simulink model "mrefrobotarm_modified_previous_y_previous_u_previous_ref_Thao"  (R2018b)
settings: Solver=FixedStepAuto  StartTime=0.0  StopTime=10  RelTol=1e-3  AbsTol=1e-6
undefined symbols (not defined in the file or in its folder): sfunxy2
libraries: neural x668, simulink x1
(part 21 of 21)

== system mrefrobotarm_modified_previous_y_previous_u_previous_ref_Thao/working_test/Layer 2/LW{2,1} ==
  "ad{2,1}" : Inport  PortDimensions=8
      mask Display: e = 0.06;c1 = [120 230 180]/255;c2 = ([120 230 180]+0)/(256+128);c3 = ([120 230 180]+128)/(256+128);patch([0 1 1 0],[0 0 1 1],c1);patch([0 1 1 1-e 1-e 0+e],[0 0 1 1-e 0+e 0+e],c2);patch([0 0 1 1-e 0+e 0+e],[0 1 1 1-e 1-e 0+e],c3);plot([0 1 1 0 0],[0 0 1 1 0]);
  "IW{2,1}(1,:)'" : Constant  Value=[1.463550825562915935762475783121772110462188720703125;1.2082669866689801363435208259033970534801483154296875;-0.6229993629461720860973628077772445976734161376953125;0.488116211879852102129007107578217983245849609375;0.84588482114214647022976123480475507676601409912109375;-1.1928719541486427768717248909524641931056976318359375;-2.057825620782761877336497491342015564441680908203125;1.5399555707144136906805442777113057672977447509765625]
      mask Display: e = 0.06;c1 = [120 150 230]/255;c2 = ([120 150 230]+0)/383;c3 = ([120 150 230]+128)/383;patch([0 1 1 0],[0 0 1 1],c1);patch([0 1 1 1-e 1-e 0+e],[0 0 1 1-e 0+e 0+e],c2);patch([0 0 1 1-e 0+e 0+e],[0 1 1 1-e 1-e 0+e],c3);plot([0 1 1 0 0],[0 0 1 1 0]);disp('weights');
  "IW{2,1}(10,:)'" : Constant  Value=[1.134018666679956321985400791163556277751922607421875;0.99363946648308232312274412834085524082183837890625;-0.54676888111817933957325976734864525496959686279296875;-0.76340597417966515880749511779868043959140777587890625;-0.9815147483076629431053561347653158009052276611328125;0.5968332702765632991059874257189221680164337158203125;1.9952854954885268501385553463478572666645050048828125;-0.92110586776434277833658370582270435988903045654296875]
      mask Display: e = 0.06;c1 = [120 150 230]/255;c2 = ([120 150 230]+0)/383;c3 = ([120 150 230]+128)/383;patch([0 1 1 0],[0 0 1 1],c1);patch([0 1 1 1-e 1-e 0+e],[0 0 1 1-e 0+e 0+e],c2);patch([0 0 1 1-e 0+e 0+e],[0 1 1 1-e 1-e 0+e],c3);plot([0 1 1 0 0],[0 0 1 1 0]);disp('weights');
  "IW{2,1}(11,:)'" : Constant  Value=[0.434041573917725853615223741144291125237941741943359375;0.16471617384395731420454467297531664371490478515625;-0.216118041022805462691991351675824262201786041259765625;2.8978280304609853601505164988338947296142578125;1.943598394902243509108075159019790589809417724609375;4.6129183278583578697862321860156953334808349609375;-0.81063433781615701345657498677610419690608978271484375;1.7612531272589067032896537057240493595600128173828125]
      mask Display: e = 0.06;c1 = [120 150 230]/255;c2 = ([120 150 230]+0)/383;c3 = ([120 150 230]+128)/383;patch([0 1 1 0],[0 0 1 1],c1);patch([0 1 1 1-e 1-e 0+e],[0 0 1 1-e 0+e 0+e],c2);patch([0 0 1 1-e 0+e 0+e],[0 1 1 1-e 1-e 0+e],c3);plot([0 1 1 0 0],[0 0 1 1 0]);disp('weights');
  "IW{2,1}(12,:)'" : Constant  Value=[1.74376096782253586781052945298142731189727783203125;0.94016947729569444458519456020439974963665008544921875;0.773288113770950413794480482465587556362152099609375;-0.72054867623120422148730312983389012515544891357421875;-0.06420804673181064459175360070730675943195819854736328125;-1.447472796373246328727191212237812578678131103515625;-0.06982005075191678733492750552613870240747928619384765625;1.6685199899347125107595957160810939967632293701171875]
      mask Display: e = 0.06;c1 = [120 150 230]/255;c2 = ([120 150 230]+0)/383;c3 = ([120 150 230]+128)/383;patch([0 1 1 0],[0 0 1 1],c1);patch([0 1 1 1-e 1-e 0+e],[0 0 1 1-e 0+e 0+e],c2);patch([0 0 1 1-e 0+e 0+e],[0 1 1 1-e 1-e 0+e],c3);plot([0 1 1 0 0],[0 0 1 1 0]);disp('weights');
  "IW{2,1}(13,:)'" : Constant  Value=[0.58611133181064423158801446334109641611576080322265625;-2.424919354117549108451612482895143330097198486328125;0.275534914445166367880091229380923323333263397216796875;-0.3179661163902725018459705097484402358531951904296875;-0.3847035616320677586799092750879935920238494873046875;-0.63707268499747760071016955407685600221157073974609375;-0.260138967832102441235520018381066620349884033203125;1.4313466678042507940205041450099088251590728759765625]
      mask Display: e = 0.06;c1 = [120 150 230]/255;c2 = ([120 150 230]+0)/383;c3 = ([120 150 230]+128)/383;patch([0 1 1 0],[0 0 1 1],c1);patch([0 1 1 1-e 1-e 0+e],[0 0 1 1-e 0+e 0+e],c2);patch([0 0 1 1-e 0+e 0+e],[0 1 1 1-e 1-e 0+e],c3);plot([0 1 1 0 0],[0 0 1 1 0]);disp('weights');
  "IW{2,1}(14,:)'" : Constant  Value=[-0.1330838655979345308555394922223058529198169708251953125;0.0807940849429321372721091165658435784280300140380859375;0.04937131990086006394502504690535715781152248382568359375;0.1369701045960752538999116723061888478696346282958984375;0.362315967016541840006738084412063471972942352294921875;0.2007900692008469933913517024848260916769504547119140625;0.357746870703516017808709648306830786168575286865234375;-1.0009625334190765943986889396910555660724639892578125]
      mask Display: e = 0.06;c1 = [120 150 230]/255;c2 = ([120 150 230]+0)/383;c3 = ([120 150 230]+128)/383;patch([0 1 1 0],[0 0 1 1],c1);patch([0 1 1 1-e 1-e 0+e],[0 0 1 1-e 0+e 0+e],c2);patch([0 0 1 1-e 0+e 0+e],[0 1 1 1-e 1-e 0+e],c3);plot([0 1 1 0 0],[0 0 1 1 0]);disp('weights');
  "IW{2,1}(15,:)'" : Constant  Value=[-1.5828584005342116736159141510142944753170013427734375;-0.34671511698060231143614373650052584707736968994140625;-0.208261551930768173956920463751885108649730682373046875;-0.71627429917518081747829228334012441337108612060546875;-1.3986327814857142382010124492808245122432708740234375;-0.033035758090816567944525417033219127915799617767333984375;1.820729591401267111194783865357749164104461669921875;-0.698698176789807501307905113208107650279998779296875]
      mask Display: e = 0.06;c1 = [120 150 230]/255;c2 = ([120 150 230]+0)/383;c3 = ([120 150 230]+128)/383;patch([0 1 1 0],[0 0 1 1],c1);patch([0 1 1 1-e 1-e 0+e],[0 0 1 1-e 0+e 0+e],c2);patch([0 0 1 1-e 0+e 0+e],[0 1 1 1-e 1-e 0+e],c3);plot([0 1 1 0 0],[0 0 1 1 0]);disp('weights');
  "IW{2,1}(16,:)'" : Constant  Value=[-1.5424575787334042775711395734106190502643585205078125;0.480620712648137493605560166543000377714633941650390625;-0.257424583228552383840082029564655385911464691162109375;-0.388965205406854419578621673281304538249969482421875;-1.523713504572799859460019433754496276378631591796875;0.39055994618596445722147336709895171225070953369140625;-2.445046000285369558469028561376035213470458984375;-1.9333998277230464157838696337421424686908721923828125]
      mask Display: e = 0.06;c1 = [120 150 230]/255;c2 = ([120 150 230]+0)/383;c3 = ([120 150 230]+128)/383;patch([0 1 1 0],[0 0 1 1],c1);patch([0 1 1 1-e 1-e 0+e],[0 0 1 1-e 0+e 0+e],c2);patch([0 0 1 1-e 0+e 0+e],[0 1 1 1-e 1-e 0+e],c3);plot([0 1 1 0 0],[0 0 1 1 0]);disp('weights');
  "IW{2,1}(17,:)'" : Constant  Value=[1.9202741200888648887001863840851001441478729248046875;3.59469018792837946563167861313559114933013916015625;1.278669491064107877065225693513639271259307861328125;0.1419885423222841669410598797185230068862438201904296875;-1.761399045758413439699552327510900795459747314453125;0.77646861010138745751163469321909360587596893310546875;-1.5057318919463986706119840164319612085819244384765625;4.2090514522541706554648044402711093425750732421875]
      mask Display: e = 0.06;c1 = [120 150 230]/255;c2 = ([120 150 230]+0)/383;c3 = ([120 150 230]+128)/383;patch([0 1 1 0],[0 0 1 1],c1);patch([0 1 1 1-e 1-e 0+e],[0 0 1 1-e 0+e 0+e],c2);patch([0 0 1 1-e 0+e 0+e],[0 1 1 1-e 1-e 0+e],c3);plot([0 1 1 0 0],[0 0 1 1 0]);disp('weights');
  "IW{2,1}(18,:)'" : Constant  Value=[2.24640861704423056011137305176816880702972412109375;0.53203674056552296978139793282025493681430816650390625;2.1547296277043468393230796209536492824554443359375;-0.9815123424716112321419814179535023868083953857421875;-0.95472145497063853891717144506401382386684417724609375;1.98605895577709556931722545414231717586517333984375;-0.034412853847981296484537239166456856764853000640869140625;5.09817173012213498139999501290731132030487060546875]
      mask Display: e = 0.06;c1 = [120 150 230]/255;c2 = ([120 150 230]+0)/383;c3 = ([120 150 230]+128)/383;patch([0 1 1 0],[0 0 1 1],c1);patch([0 1 1 1-e 1-e 0+e],[0 0 1 1-e 0+e 0+e],c2);patch([0 0 1 1-e 0+e 0+e],[0 1 1 1-e 1-e 0+e],c3);plot([0 1 1 0 0],[0 0 1 1 0]);disp('weights');
  "IW{2,1}(19,:)'" : Constant  Value=[0.7794520854145703392390487351804040372371673583984375;-1.895929436985962279749173831078223884105682373046875;-1.7189894476246034837885190427186898887157440185546875;-0.6837047167167085159888983980636112391948699951171875;0.34353814452782016619636351606459356844425201416015625;-4.143145140083309030387681559659540653228759765625;2.2429389993183068696680493303574621677398681640625;3.682068418408167786992635228671133518218994140625]
      mask Display: e = 0.06;c1 = [120 150 230]/255;c2 = ([120 150 230]+0)/383;c3 = ([120 150 230]+128)/383;patch([0 1 1 0],[0 0 1 1],c1);patch([0 1 1 1-e 1-e 0+e],[0 0 1 1-e 0+e 0+e],c2);patch([0 0 1 1-e 0+e 0+e],[0 1 1 1-e 1-e 0+e],c3);plot([0 1 1 0 0],[0 0 1 1 0]);disp('weights');
  "IW{2,1}(2,:)'" : Constant  Value=[1.0654566777175968894653124152682721614837646484375;0.002032816601710635100175306178016398916952311992645263671875;2.1595672663571736649146259878762066364288330078125;0.92280763301808221843458568400819785892963409423828125;1.768096961470302375118990312330424785614013671875;1.6041779041884136614015687882783822715282440185546875;0.7628890513396715533644965034909546375274658203125;-3.6541749563162664315996153163723647594451904296875]
      mask Display: e = 0.06;c1 = [120 150 230]/255;c2 = ([120 150 230]+0)/383;c3 = ([120 150 230]+128)/383;patch([0 1 1 0],[0 0 1 1],c1);patch([0 1 1 1-e 1-e 0+e],[0 0 1 1-e 0+e 0+e],c2);patch([0 0 1 1-e 0+e 0+e],[0 1 1 1-e 1-e 0+e],c3);plot([0 1 1 0 0],[0 0 1 1 0]);disp('weights');
  "IW{2,1}(20,:)'" : Constant  Value=[-0.103154969350188807641899302325327880680561065673828125;2.252970323340981462223453490878455340862274169921875;-0.96843329729804239480728256239672191441059112548828125;-1.902193396943337777571514379815198481082916259765625;0.366418820839169268044344107693177647888660430908203125;-2.270850899561910551938126445747911930084228515625;-1.3039885334908654090924073898349888622760772705078125;0.50925510859634848248589378272299654781818389892578125]
      mask Display: e = 0.06;c1 = [120 150 230]/255;c2 = ([120 150 230]+0)/383;c3 = ([120 150 230]+128)/383;patch([0 1 1 0],[0 0 1 1],c1);patch([0 1 1 1-e 1-e 0+e],[0 0 1 1-e 0+e 0+e],c2);patch([0 0 1 1-e 0+e 0+e],[0 1 1 1-e 1-e 0+e],c3);plot([0 1 1 0 0],[0 0 1 1 0]);disp('weights');
  "IW{2,1}(3,:)'" : Constant  Value=[-0.66339214473495022872384652146138250827789306640625;-0.222233047173612863200986566880601458251476287841796875;-0.81637664684851396490472552613937295973300933837890625;-0.668398882047606779366333284997381269931793212890625;1.9962758949163597055331820229184813797473907470703125;-0.27992544835338295516891093939193524420261383056640625;-0.94498420997124610298811830944032408297061920166015625;0.337485237137902682746926075196824967861175537109375]
      mask Display: e = 0.06;c1 = [120 150 230]/255;c2 = ([120 150 230]+0)/383;c3 = ([120 150 230]+128)/383;patch([0 1 1 0],[0 0 1 1],c1);patch([0 1 1 1-e 1-e 0+e],[0 0 1 1-e 0+e 0+e],c2);patch([0 0 1 1-e 0+e 0+e],[0 1 1 1-e 1-e 0+e],c3);plot([0 1 1 0 0],[0 0 1 1 0]);disp('weights');
  "IW{2,1}(4,:)'" : Constant  Value=[-2.20465810888284341473308813874609768390655517578125;2.584547994441787732711190983536653220653533935546875;-1.0462844726166229403219176674610935151576995849609375;3.5487772443023413160290147061459720134735107421875;-0.182806955450451835698544300612411461770534515380859375;0.235620634411733476110129004155169241130352020263671875;-2.22555439962967671618798704002983868122100830078125;-2.11305052916475322177802809164859354496002197265625]
      mask Display: e = 0.06;c1 = [120 150 230]/255;c2 = ([120 150 230]+0)/383;c3 = ([120 150 230]+128)/383;patch([0 1 1 0],[0 0 1 1],c1);patch([0 1 1 1-e 1-e 0+e],[0 0 1 1-e 0+e 0+e],c2);patch([0 0 1 1-e 0+e 0+e],[0 1 1 1-e 1-e 0+e],c3);plot([0 1 1 0 0],[0 0 1 1 0]);disp('weights');
  "IW{2,1}(5,:)'" : Constant  Value=[1.31774560984433275478977520833723247051239013671875;-0.360000305828590716483716960283345542848110198974609375;-0.311464151704573255496910633155493997037410736083984375;-1.0610633589393507758558143905247561633586883544921875;0.6481786802746196674007705951225943863391876220703125;1.9720589174498897033771527276257984340190887451171875;0.7658460266185020959284202035632915794849395751953125;3.26223001214720564888693843386135995388031005859375]
      mask Display: e = 0.06;c1 = [120 150 230]/255;c2 = ([120 150 230]+0)/383;c3 = ([120 150 230]+128)/383;patch([0 1 1 0],[0 0 1 1],c1);patch([0 1 1 1-e 1-e 0+e],[0 0 1 1-e 0+e 0+e],c2);patch([0 0 1 1-e 0+e 0+e],[0 1 1 1-e 1-e 0+e],c3);plot([0 1 1 0 0],[0 0 1 1 0]);disp('weights');
  "IW{2,1}(6,:)'" : Constant  Value=[0.7726601955585319370101160529884509742259979248046875;0.58889404743400375341622066116542555391788482666015625;-1.0756676160532527841695582537795417010784149169921875;-1.197073377238570213165758104878477752208709716796875;0.030446979813859798014163970947265625;-0.4042833226405779800671780321863479912281036376953125;0.42715808275051048159554056837805546820163726806640625;-0.6995334276770768244801956825540401041507720947265625]
      mask Display: e = 0.06;c1 = [120 150 230]/255;c2 = ([120 150 230]+0)/383;c3 = ([120 150 230]+128)/383;patch([0 1 1 0],[0 0 1 1],c1);patch([0 1 1 1-e 1-e 0+e],[0 0 1 1-e 0+e 0+e],c2);patch([0 0 1 1-e 0+e 0+e],[0 1 1 1-e 1-e 0+e],c3);plot([0 1 1 0 0],[0 0 1 1 0]);disp('weights');
  "IW{2,1}(7,:)'" : Constant  Value=[-0.7725295931807278915215420056483708322048187255859375;-2.173121115889052656910962468828074634075164794921875;-0.1818589726845724896531208969463477842509746551513671875;0.637043349560801441811008771765045821666717529296875;-2.165436289512435497073283841018564999103546142578125;2.37097135712689777164996485225856304168701171875;2.277406878831848668909287880524061620235443115234375;-1.4636931671188297965358060537255369126796722412109375]
      mask Display: e = 0.06;c1 = [120 150 230]/255;c2 = ([120 150 230]+0)/383;c3 = ([120 150 230]+128)/383;patch([0 1 1 0],[0 0 1 1],c1);patch([0 1 1 1-e 1-e 0+e],[0 0 1 1-e 0+e 0+e],c2);patch([0 0 1 1-e 0+e 0+e],[0 1 1 1-e 1-e 0+e],c3);plot([0 1 1 0 0],[0 0 1 1 0]);disp('weights');
  "IW{2,1}(8,:)'" : Constant  Value=[2.6381111188624846164429982309229671955108642578125;2.13100131299981665478071590769104659557342529296875;-1.6010659213930111821611035338719375431537628173828125;-0.046612756831267587731559842723072506487369537353515625;1.1429029499162701721814983102376572787761688232421875;-0.6486750417208211327846356653026305139064788818359375;1.9735437620485793974722810162347741425037384033203125;1.296947831419701824273715828894637525081634521484375]
      mask Display: e = 0.06;c1 = [120 150 230]/255;c2 = ([120 150 230]+0)/383;c3 = ([120 150 230]+128)/383;patch([0 1 1 0],[0 0 1 1],c1);patch([0 1 1 1-e 1-e 0+e],[0 0 1 1-e 0+e 0+e],c2);patch([0 0 1 1-e 0+e 0+e],[0 1 1 1-e 1-e 0+e],c3);plot([0 1 1 0 0],[0 0 1 1 0]);disp('weights');
  "IW{2,1}(9,:)'" : Constant  Value=[0.389378863511709749634093213899177499115467071533203125;-3.044010638669162549518887317390181124210357666015625;2.170328036093251089511113605112768709659576416015625;3.090312720034663840351640828885138034820556640625;-1.84388163895774592759835286415182054042816162109375;-0.35509810169707411997563895056373439729213714599609375;-2.31952597061908960540677071548998355865478515625;-1.2086983328395906056584863108582794666290283203125]
      mask Display: e = 0.06;c1 = [120 150 230]/255;c2 = ([120 150 230]+0)/383;c3 = ([120 150 230]+128)/383;patch([0 1 1 0],[0 0 1 1],c1);patch([0 1 1 1-e 1-e 0+e],[0 0 1 1-e 0+e 0+e],c2);patch([0 0 1 1-e 0+e 0+e],[0 1 1 1-e 1-e 0+e],c3);plot([0 1 1 0 0],[0 0 1 1 0]);disp('weights');
  Mux : Mux  Inputs=20
      mask Display: e = 0.06;c1 = [120 150 230]/255;c2 = ([120 150 230]+0)/383;c3 = ([120 150 230]+128)/383;patch([0 1 1 0],[0 0 1 1],c1);patch([0 1 1 1-e 1-e 0+e],[0 0 1 1-e 0+e 0+e],c2);patch([0 0 1 1-e 0+e 0+e],[0 1 1 1-e 1-e 0+e],c3);plot([0 1 1 0 0],[0 0 1 1 0]);disp('Mux');
  dotprod{1..20} (20 alike) : neural/Weight Functions/dotprod
  "lz{2,1}" : Outport
      mask Display: e = 0.06;c1 = [120 230 180]/255;c2 = ([120 230 180]+0)/(256+128);c3 = ([120 230 180]+128)/(256+128);patch([0 1 1 0],[0 0 1 1],c1);patch([0 1 1 1-e 1-e 0+e],[0 0 1 1-e 0+e 0+e],c2);patch([0 0 1 1-e 0+e 0+e],[0 1 1 1-e 1-e 0+e],c3);plot([0 1 1 0 0],[0 0 1 1 0]);
  wires:
  "IW{2,1}(1,:)'"/1 -> dotprod1/1
  "ad{2,1}"/1 -> dotprod1/2, dotprod2/2, dotprod3/2, dotprod4/2, dotprod5/2, dotprod6/2, dotprod7/2, dotprod8/2, dotprod9/2, dotprod10/2, dotprod11/2, dotprod12/2, dotprod13/2, dotprod14/2, dotprod15/2, dotprod16/2, dotprod17/2, dotprod18/2, dotprod19/2, dotprod20/2
  dotprod1/1 -> Mux/1
  "IW{2,1}(2,:)'"/1 -> dotprod2/1
  dotprod2/1 -> Mux/2
  "IW{2,1}(3,:)'"/1 -> dotprod3/1
  dotprod3/1 -> Mux/3
  "IW{2,1}(4,:)'"/1 -> dotprod4/1
  dotprod4/1 -> Mux/4
  "IW{2,1}(5,:)'"/1 -> dotprod5/1
  dotprod5/1 -> Mux/5
  "IW{2,1}(6,:)'"/1 -> dotprod6/1
  dotprod6/1 -> Mux/6
  "IW{2,1}(7,:)'"/1 -> dotprod7/1
  dotprod7/1 -> Mux/7
  "IW{2,1}(8,:)'"/1 -> dotprod8/1
  dotprod8/1 -> Mux/8
  "IW{2,1}(9,:)'"/1 -> dotprod9/1
  dotprod9/1 -> Mux/9
  "IW{2,1}(10,:)'"/1 -> dotprod10/1
  dotprod10/1 -> Mux/10
  "IW{2,1}(11,:)'"/1 -> dotprod11/1
  dotprod11/1 -> Mux/11
  "IW{2,1}(12,:)'"/1 -> dotprod12/1
  dotprod12/1 -> Mux/12
  "IW{2,1}(13,:)'"/1 -> dotprod13/1
  dotprod13/1 -> Mux/13
  "IW{2,1}(14,:)'"/1 -> dotprod14/1
  dotprod14/1 -> Mux/14
  "IW{2,1}(15,:)'"/1 -> dotprod15/1
  dotprod15/1 -> Mux/15
  "IW{2,1}(16,:)'"/1 -> dotprod16/1
  dotprod16/1 -> Mux/16
  "IW{2,1}(17,:)'"/1 -> dotprod17/1
  dotprod17/1 -> Mux/17
  "IW{2,1}(18,:)'"/1 -> dotprod18/1
  dotprod18/1 -> Mux/18
  "IW{2,1}(19,:)'"/1 -> dotprod19/1
  dotprod19/1 -> Mux/19
  "IW{2,1}(20,:)'"/1 -> dotprod20/1
  dotprod20/1 -> Mux/20
  Mux/1 -> "lz{2,1}"/1

== system mrefrobotarm_modified_previous_y_previous_u_previous_ref_Thao/working_test/Layer 3/Delays 1 ==
  "p{3}" : Inport  PortDimensions=20
      mask Display: e = 0.06;c1 = [120 230 180]/255;c2 = ([120 230 180]+0)/(256+128);c3 = ([120 230 180]+128)/(256+128);patch([0 1 1 0],[0 0 1 1],c1);patch([0 1 1 1-e 1-e 0+e],[0 0 1 1-e 0+e 0+e],c2);patch([0 0 1 1-e 0+e 0+e],[0 1 1 1-e 1-e 0+e],c3);plot([0 1 1 0 0],[0 0 1 1 0]);
  mux : Mux  Inputs=1
      mask Display: e = 0.06;c1 = [120 150 230]/255;c2 = ([120 150 230]+0)/383;c3 = ([120 150 230]+128)/383;patch([0 1 1 0],[0 0 1 1],c1);patch([0 1 1 1-e 1-e 0+e],[0 0 1 1-e 0+e 0+e],c2);patch([0 0 1 1-e 0+e 0+e],[0 1 1 1-e 1-e 0+e],c3);plot([0 1 1 0 0],[0 0 1 1 0]);disp('Mux')
  "pd{3,2}" : Outport
      mask Display: e = 0.06;c1 = [120 230 180]/255;c2 = ([120 230 180]+0)/(256+128);c3 = ([120 230 180]+128)/(256+128);patch([0 1 1 0],[0 0 1 1],c1);patch([0 1 1 1-e 1-e 0+e],[0 0 1 1-e 0+e 0+e],c2);patch([0 0 1 1-e 0+e 0+e],[0 1 1 1-e 1-e 0+e],c3);plot([0 1 1 0 0],[0 0 1 1 0]);
  wires:
  "p{3}"/1 -> mux/1
  mux/1 -> "pd{3,2}"/1

== system mrefrobotarm_modified_previous_y_previous_u_previous_ref_Thao/working_test/Layer 3/LW{3,2} ==
  "ad{3,2}" : Inport  PortDimensions=20
      mask Display: e = 0.06;c1 = [120 230 180]/255;c2 = ([120 230 180]+0)/(256+128);c3 = ([120 230 180]+128)/(256+128);patch([0 1 1 0],[0 0 1 1],c1);patch([0 1 1 1-e 1-e 0+e],[0 0 1 1-e 0+e 0+e],c2);patch([0 0 1 1-e 0+e 0+e],[0 1 1 1-e 1-e 0+e],c3);plot([0 1 1 0 0],[0 0 1 1 0]);
  "IW{3,2}(1,:)'" : Constant  Value=[0.03553375757208938889863958365822327323257923126220703125;-0.1695200442229983506248203184441081248223781585693359375;0.056376011217140677145298610639656544663012027740478515625;0.095613046029798087754869584387051872909069061279296875;-0.380472867925660984678160048133577220141887664794921875;0.1588426820544598105922062813988304696977138519287109375;0.00632939270960307560909274826599357766099274158477783203125;-0.0276922201875561373174416956999266403727233409881591796875;0.102556443455339596493303133684094063937664031982421875;-0.5356637743242409488431121644680388271808624267578125;0.0547402153952234182821001695629092864692211151123046875;-0.042467052158223279889615042748118867166340351104736328125;0.67093156298297629280824594388832338154315948486328125;2.683757086825995230583430384285748004913330078125;-0.11889956662100518991476150176822557114064693450927734375;-0.0312957872856202412581438920824439264833927154541015625;-0.1077738407852244229001570374748553149402141571044921875;0.1283284583454132044000317591780913062393665313720703125;-0.09002225517494165385468107842825702391564846038818359375;0.0527813037228504755571378836975782178342342376708984375]
      mask Display: e = 0.06;c1 = [120 150 230]/255;c2 = ([120 150 230]+0)/383;c3 = ([120 150 230]+128)/383;patch([0 1 1 0],[0 0 1 1],c1);patch([0 1 1 1-e 1-e 0+e],[0 0 1 1-e 0+e 0+e],c2);patch([0 0 1 1-e 0+e 0+e],[0 1 1 1-e 1-e 0+e],c3);plot([0 1 1 0 0],[0 0 1 1 0]);disp('weights');
  Mux : Mux  Inputs=1
      mask Display: e = 0.06;c1 = [120 150 230]/255;c2 = ([120 150 230]+0)/383;c3 = ([120 150 230]+128)/383;patch([0 1 1 0],[0 0 1 1],c1);patch([0 1 1 1-e 1-e 0+e],[0 0 1 1-e 0+e 0+e],c2);patch([0 0 1 1-e 0+e 0+e],[0 1 1 1-e 1-e 0+e],c3);plot([0 1 1 0 0],[0 0 1 1 0]);disp('Mux');
  dotprod1 : neural/Weight Functions/dotprod
  "lz{3,2}" : Outport
      mask Display: e = 0.06;c1 = [120 230 180]/255;c2 = ([120 230 180]+0)/(256+128);c3 = ([120 230 180]+128)/(256+128);patch([0 1 1 0],[0 0 1 1],c1);patch([0 1 1 1-e 1-e 0+e],[0 0 1 1-e 0+e 0+e],c2);patch([0 0 1 1-e 0+e 0+e],[0 1 1 1-e 1-e 0+e],c3);plot([0 1 1 0 0],[0 0 1 1 0]);
  wires:
  "IW{3,2}(1,:)'"/1 -> dotprod1/1
  "ad{3,2}"/1 -> dotprod1/2
  dotprod1/1 -> Mux/1
  Mux/1 -> "lz{3,2}"/1
